simulink model "modele_cl3"  (R2026a)
settings: Solver=VariableStepAuto

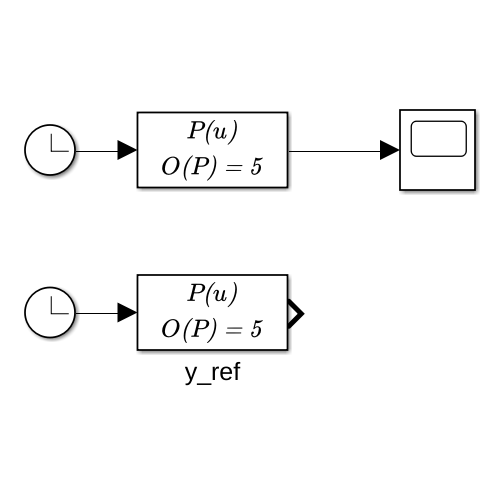
[thumbnail: Simulink's stored preview of the top-level diagram]
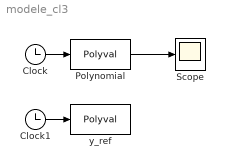
== system modele_cl3 ==
  Clock : Clock
  Clock1 : Clock
  Polynomial : Polyval  Coefs=[0, 0, -2e-3, 2e-3, 0.1, 2.32e-3]
  Scope : Scope
      settings: ActiveDisplayYMinimum=-0.93622400000000017  ActiveDisplayYMaximum=0.44921599999999995
  y_ref : Polyval  Coefs=[0, -1e-4, -2e-4, 4.89e-2, 2.3e-3, -1e-3]
  wires:
  Clock/1 -> Polynomial/1
  Polynomial/1 -> Scope/1
  Clock1/1 -> y_ref/1
